simulink model "half_bridge_project"  (R2020b)
settings: Solver=VariableStepAuto  StartTime=0.0  StopTime=2  RelTol=1e-3
libraries: powerlib x9, powerlib_meascontrol x1
settings Model: Creator=pouya  LastModifiedBy=mcapuano

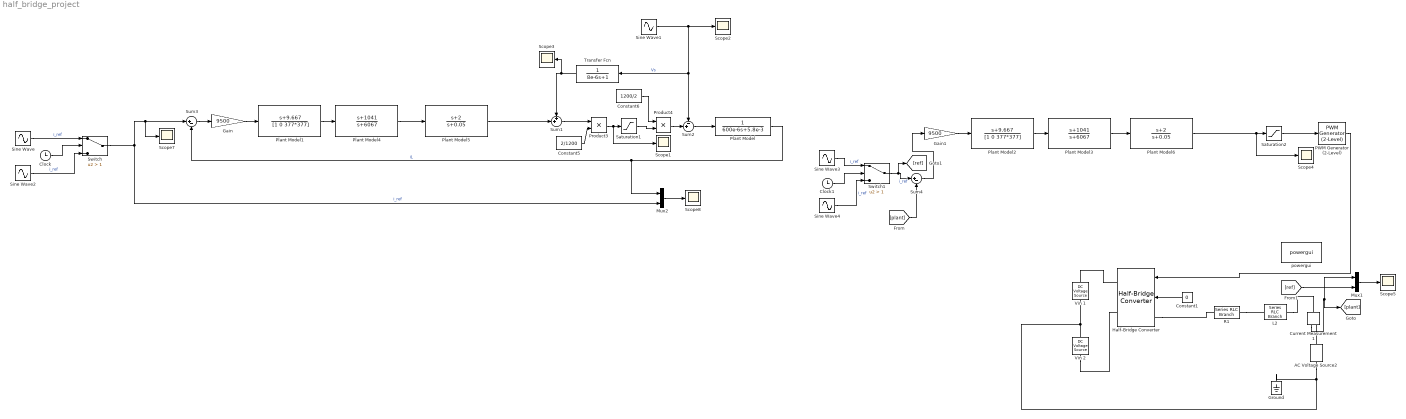
== system half_bridge_project ==
  AC Voltage Source2 : powerlib/Electrical Sources/AC Voltage Source  Amplitude=400  Phase=-60  Frequency=60  SampleTime=0  Measurements=None  BusType=swing  Pref=10e3  Qref=0  Qmin=-inf  Qmax=+inf
  Clock : Clock
  Clock1 : Clock
  Constant1 : Constant  Value=0
  Constant5 : Constant  Value=2/1200
  Constant6 : Constant  Value=1200/2
  Current Measurement1 : powerlib/Measurements/Current Measurement  PhasorSimulation=off  OutputType=Complex  PSBequivalent=0
  Gain : Gain  Gain=9500
  Gain1 : Gain  Gain=9500
  Ground : powerlib/Elements/Ground  LConnTagsString=a
  Half-Bridge Converter : powerlib/Power Electronics/Half-Bridge Converter  ModelType=Switching devices  Ron=1e-3  Rs=1e6  Cs=inf  Vforward=[0,0]  Ron_Diode=1e-3  Rs_Diode=1e6  Cs_Diode=inf  Vf_Diode=1e-3  Rs_CurrentSource=inf
      settings: SourceProductBaseCode=PS
  L2 : powerlib/Elements/Series RLC Branch  LConnTagsString=__new0  RConnTagsString=__new0  BranchType=L  Resistance=1e-4  Inductance=600e-6  SetiL0=on  InitialCurrent=.1  Capacitance=30e-6  Setx0=off  InitialVoltage=150  Measurements=None
  Mux1 : Mux  Inputs=2
  Mux2 : Mux  Inputs=2
  PWM Generator (2-Level) : powerlib_meascontrol/Pulse & Signal Generators/PWM Generator (2-Level)  ModulatorType=Single-phase half-bridge (2 pulses)  ModulatorMode=Unsynchronized  Fc=1620  Pc=90  nF=27  MinMax="[ -1  1 ]"  SamplingTechnique=Natural  ModulatingSignals=off  m=0.8  Freq=60  Phase=0  Ts=0  ShowCarrierOutport=off
  Plant Model : TransferFcn  Denominator=[600e-6 5.8e-3]
  Plant Model1 : TransferFcn  Numerator=[1 9.667]  Denominator=[1 0 377*377]
  Plant Model2 : TransferFcn  Numerator=[1 9.667]  Denominator=[1 0 377*377]
  Plant Model3 : TransferFcn  Numerator=[1 1041]  Denominator=[1 6067]
  Plant Model4 : TransferFcn  Numerator=[1 1041]  Denominator=[1 6067]
  Plant Model5 : TransferFcn  Numerator=[1 2]  Denominator=[1 0.05]
  Plant Model6 : TransferFcn  Numerator=[1 2]  Denominator=[1 0.05]
  Product3 : Product
  Product4 : Product
  R1 : powerlib/Elements/Series RLC Branch  LConnTagsString=__new0  RConnTagsString=__new0  BranchType=R  Resistance=5.8e-3  Inductance=200e-6  SetiL0=off  InitialCurrent=0  Capacitance=400e-6  Setx0=off  InitialVoltage=0  Measurements=None
  Saturation1 : Saturate  UpperLimit=1  LowerLimit=-1
  Saturation2 : Saturate  UpperLimit=1  LowerLimit=-1
  Scope{1..5,7..8} (7 alike) : Scope
  Sine Wave : Sin  Amplitude=150  Frequency=377  Phase=-pi/3  SampleTime=0
  Sine Wave1 : Sin  Amplitude=400  Frequency=377  Phase=-pi/3  SampleTime=0
  Sine Wave2 : Sin  Amplitude=100  Frequency=377  Phase=-pi/3  SampleTime=0
  Sine Wave3 : Sin  Amplitude=150  Frequency=377  Phase=-pi/3  SampleTime=0
  Sine Wave4 : Sin  Amplitude=100  Frequency=377  Phase=-pi/3  SampleTime=0
  Sum1 : Sum  Inputs=++|
  Sum2 : Sum  Inputs=-+|
  Sum3 : Sum  Inputs=|+-
  Sum4 : Sum  Inputs=|+-
  Switch : Switch  Criteria=u2 > Threshold  Threshold=1
  Switch1 : Switch  Criteria=u2 > Threshold  Threshold=1
  Transfer Fcn : TransferFcn  Denominator=[8e-6 1]
  Vin 1 : powerlib/Electrical Sources/DC Voltage Source  Amplitude=600  Measurements=None
  Vin 2 : powerlib/Electrical Sources/DC Voltage Source  Amplitude=600  Measurements=None
  powergui : powerlib/powergui  Priority=1  SimulationMode=Continuous  SampleTime=50e-6  frequency=60  Iterations=50  frequencyindice=0  Pbase=100e6  ErrMax=1e-4  UnitsV=kV  UnitsW=MW  buscounter=0  FunctionMessages=off  echomessages=off  EnableUseOfTLC=off  CurrentSourceSwitches=off  DisableSnubberDevices=off  DisableRonSwitches=off  DisableVfSwitches=off  DisplayEquations=off  AutomaticDiscreteSolvers=off  SolverType=Tustin/Backward Euler (TBE)  Interpol=off  ExternalGateDelay=off  methode=off  Ts=100  x0status=blocks  SPID=on  SwTol=0  HookPort=off  NonlinearTolerance=1e-4  nMaxIteration=100  ContinueOnMaxIteration=off  RestoreLinks=warning  ResistiveCurrentMeasurement=off  Frange=[0:2:500]  Ylog=off  Xlog=on  ShowGrid=off  save=off  variable=ZData  structure=0  ZoomFFT=off  StartTime=0.0  cycles=1  DisplayStyle=1  fundamental=60  FreqAxis=off  MaxFrequency=1000  frequencyindicesteady=1  RmsSteady=1  display=off
  wires:
  Sum2/1 -> Plant Model/1
  Constant5/1 -> Product3/2
  Product3/1 -> Scope1/1, Saturation1/1
  Switch/1 -> Mux2/2, Scope7/1, Sum3/1  "i_ref"
  Plant Model/1 -> Mux2/1, Sum3/2  "iL"
  Sum3/1 -> Gain/1
  Mux2/1 -> Scope8/1
  Constant6/1 -> Product4/1
  Saturation1/1 -> Product4/2
  Sum1/1 -> Product3/1
  Product4/1 -> Sum2/2
  Transfer Fcn/1 -> Sum1/1, Scope3/1
  Sine Wave1/1 -> Scope2/1, Sum2/1, Transfer Fcn/1  "Vs"
  Gain/1 -> Plant Model1/1
  Plant Model1/1 -> Plant Model4/1
  Plant Model4/1 -> Plant Model5/1
  Plant Model5/1 -> Sum1/2
  Sine Wave2/1 -> Switch/3  "i_ref"
  Sine Wave/1 -> Switch/1  "i_ref"
  Clock/1 -> Switch/2
  Gain1/1 -> Plant Model2/1
  Plant Model2/1 -> Plant Model3/1
  Sum4/1 -> Gain1/1
  Plant Model3/1 -> Plant Model6/1
  Plant Model6/1 -> Scope4/1, Saturation2/1
  Sine Wave4/1 -> Switch1/3  "i_ref"
  Clock1/1 -> Switch1/2
  Sine Wave3/1 -> Switch1/1  "i_ref"
  Switch1/1 -> [ref], Sum4/1  "i_ref"
  [plant] -> Sum4/2
  Current Measurement1/1 -> Mux1/1, [plant]
  Mux1/1 -> Scope5/1
  [ref] -> Mux1/2
  Constant1/1 -> Half-Bridge Converter/2
  Saturation2/1 -> PWM Generator (2-Level)/1
  PWM Generator (2-Level)/1 -> Half-Bridge Converter/1
  connections:
  R1/RConn1 -- L2/LConn1
  Vin 1/RConn1 -- Half-Bridge Converter/RConn1
  Vin 2/LConn1 -- Half-Bridge Converter/RConn2
  Vin 2/RConn1 -- AC Voltage Source2/LConn1 -- Ground/LConn1 -- Vin 1/LConn1
  L2/RConn1 -- Current Measurement1/LConn1
  Half-Bridge Converter/LConn1 -- R1/LConn1
  AC Voltage Source2/RConn1 -- Current Measurement1/RConn1
